simulink model "VK"  (R2022b)
settings: Solver=ode1  StartTime=0.0  StopTime=240  FixedStep=0.01  RelTol=1e-3
undefined symbols (not defined in the file or in its folder): F, Light, MIL, Newton, Raphson, sigbuilder_block
libraries: simulink x3, aerolibwind2 x2, aerolibutil x1, sharedtransform x1
settings Model: Creator=jmira  LastModifiedBy=armando
settings DebuggingCC: UnconnectedInputMsg=warning  UnconnectedOutputMsg=warning  UnconnectedLineMsg=warning
settings ModelReferenceCC: EnableRefExpFcnMdlSchedulingChecks=on
settings RTWCC: DLArmComputeVersion=19.05

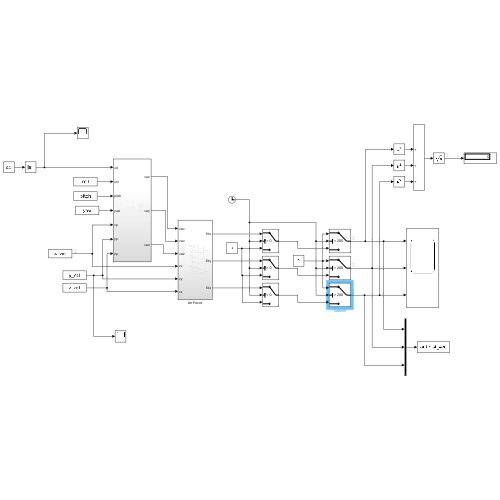
[thumbnail: Simulink's stored preview of the top-level diagram]
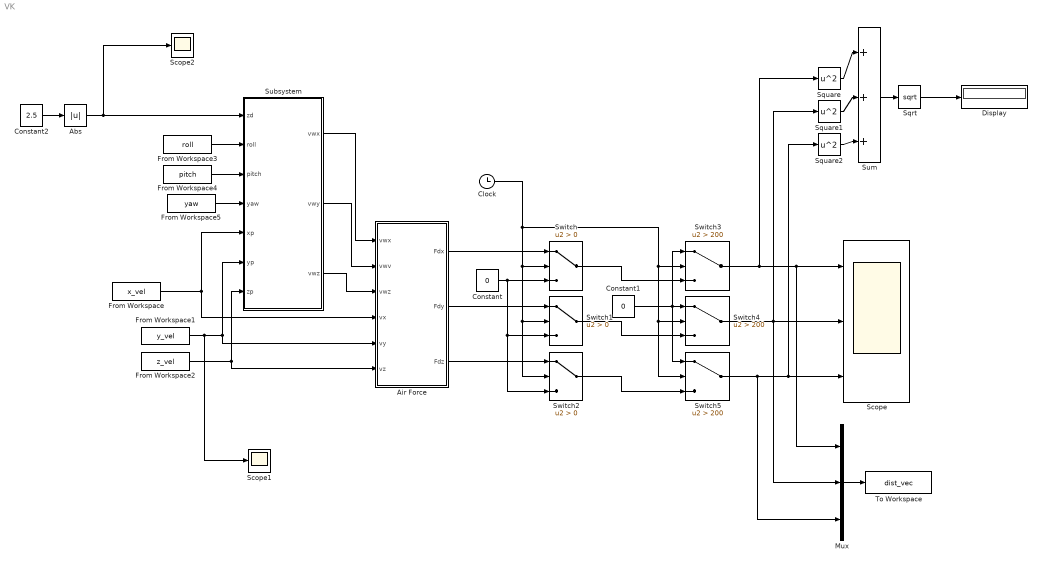
== system VK ==
  Abs : Abs  SaturateOnIntegerOverflow=off
  Air Force : Subsystem
  Clock : Clock
  Constant : Constant  Value=0
  Constant1 : Constant  Value=0
  Constant2 : Constant  Value=2.5
  Display : Display
  From Workspace : FromWorkspace  VariableName=x_vel  SampleTime=0.01
  From Workspace1 : FromWorkspace  VariableName=y_vel  SampleTime=0.01
  From Workspace2 : FromWorkspace  VariableName=z_vel  SampleTime=0.01
  From Workspace3 : FromWorkspace  VariableName=roll  SampleTime=0.01
  From Workspace4 : FromWorkspace  VariableName=pitch  SampleTime=0.01
  From Workspace5 : FromWorkspace  VariableName=yaw  SampleTime=0.01
  Mux : Mux  Inputs=3
  Scope : Scope  NumInputPorts=3
  Scope1 : Scope
  Scope2 : Scope
  Sqrt : Sqrt
  Square : Math  Operator=square
  Square1 : Math  Operator=square
  Square2 : Math  Operator=square
  Subsystem : Subsystem
  Sum : Sum  Inputs=|+++
  Switch : Switch  Criteria=u2 > Threshold  SaturateOnIntegerOverflow=off  InputSameDT=off
  Switch1 : Switch  Criteria=u2 > Threshold  SaturateOnIntegerOverflow=off  InputSameDT=off
  Switch2 : Switch  Criteria=u2 > Threshold  SaturateOnIntegerOverflow=off  InputSameDT=off
  Switch3 : Switch  Criteria=u2 > Threshold  Threshold=200  SaturateOnIntegerOverflow=off  InputSameDT=off
  Switch4 : Switch  Criteria=u2 > Threshold  Threshold=200  SaturateOnIntegerOverflow=off  InputSameDT=off
  Switch5 : Switch  Criteria=u2 > Threshold  Threshold=200  SaturateOnIntegerOverflow=off  InputSameDT=off
  To Workspace : ToWorkspace  VariableName=dist_vec  SampleTime=-1
      settings: Save2DSignal=2-D array (concatenate along first dimension)
  wires:
  Abs/1 -> Scope2/1, Subsystem/1(zd)
  Subsystem/1(vwx) -> Air Force/1(vwx)
  From Workspace/1 -> Air Force/4(vx), Subsystem/5(xp)
  Subsystem/3(vwz) -> Air Force/3(vwz)
  From Workspace1/1 -> Scope1/1, Air Force/5(vy), Subsystem/6(yp)
  Subsystem/2(vwy) -> Air Force/2(vwv)
  From Workspace2/1 -> Air Force/6(vz), Subsystem/7(zp)
  From Workspace3/1 -> Subsystem/2(roll)
  From Workspace4/1 -> Subsystem/3(pitch)
  From Workspace5/1 -> Subsystem/4(yaw)
  Mux/1 -> To Workspace/1
  Air Force/1(Fdx) -> Switch/1
  Clock/1 -> Switch5/2, Switch4/2, Switch3/2, Switch2/2, Switch1/2, Switch/2
  Constant/1 -> Switch2/3, Switch1/3, Switch/3
  Air Force/2(Fdy) -> Switch1/1
  Air Force/3(Fdz) -> Switch2/1
  Switch/1 -> Switch3/3
  Constant1/1 -> Switch5/1, Switch3/1, Switch4/1
  Switch1/1 -> Switch4/3
  Switch2/1 -> Switch5/3
  Switch3/1 -> Square/1, Mux/1, Scope/1
  Switch4/1 -> Square1/1, Mux/2, Scope/2
  Switch5/1 -> Mux/3, Square2/1, Scope/3
  Constant2/1 -> Abs/1
  Square/1 -> Sum/1
  Square2/1 -> Sum/3
  Square1/1 -> Sum/2
  Sum/1 -> Sqrt/1
  Sqrt/1 -> Display/1

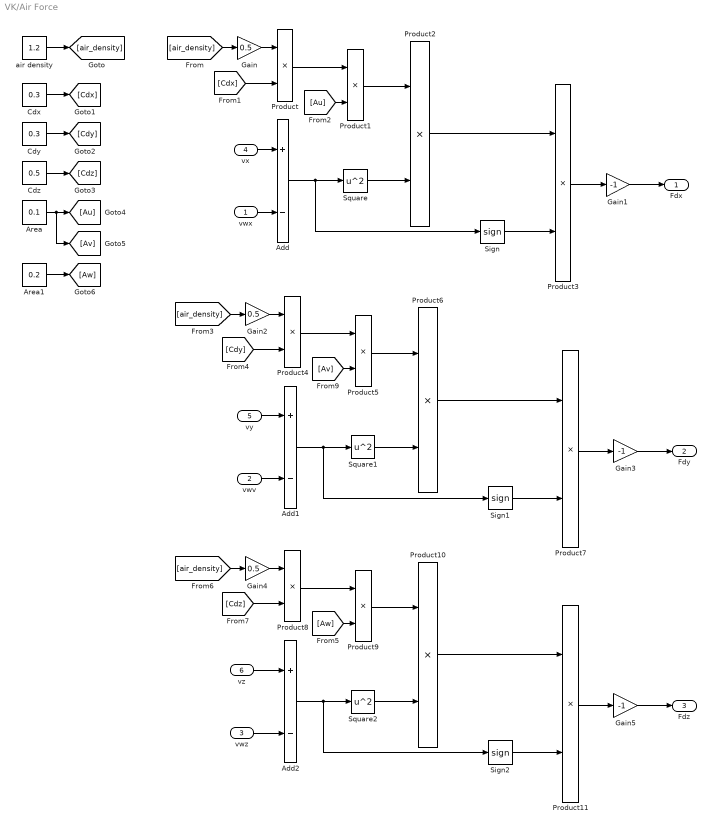
== system VK/Air Force ==
  vwx : Inport
  vwv : Inport  Port=2
  vwz : Inport  Port=3
  vx : Inport  Port=4
  vy : Inport  Port=5
  vz : Inport  Port=6
  Add : Sum  Inputs=+-
  Add1 : Sum  Inputs=+-
  Add2 : Sum  Inputs=+-
  Area : Constant  Value=0.1
  Area1 : Constant  Value=0.2
  Cdx : Constant  Value=0.3
  Cdy : Constant  Value=0.3
  Cdz : Constant  Value=0.5
  Gain : Gain  Gain=0.5
  Gain1 : Gain  Gain=-1
  Gain2 : Gain  Gain=0.5
  Gain3 : Gain  Gain=-1
  Gain4 : Gain  Gain=0.5
  Gain5 : Gain  Gain=-1
  Product{,1..11} (12 alike) : Product
  Sign : Signum
  Sign1 : Signum
  Sign2 : Signum
  Square : Math  Operator=square
  Square1 : Math  Operator=square
  Square2 : Math  Operator=square
  air density : Constant  Value=1.2
  Fdx : Outport
  Fdy : Outport  Port=2
  Fdz : Outport  Port=3
  wires:
  air density/1 -> [air_density]
  [air_density] -> Gain/1
  Cdx/1 -> [Cdx]
  Cdy/1 -> [Cdy]
  Cdz/1 -> [Cdz]
  Gain/1 -> Product/1
  [Cdx] -> Product/2
  Area/1 -> [Av], [Au]
  Product/1 -> Product1/1
  [Au] -> Product1/2
  Product1/1 -> Product2/1
  Square/1 -> Product2/2
  Add/1 -> Sign/1, Square/1
  vx/1 -> Add/1
  vwx/1 -> Add/2
  Product2/1 -> Product3/1
  Sign/1 -> Product3/2
  Product3/1 -> Gain1/1
  Gain1/1 -> Fdx/1
  Gain3/1 -> Fdy/1
  Product7/1 -> Gain3/1
  Sign1/1 -> Product7/2
  Product6/1 -> Product7/1
  vwv/1 -> Add1/2
  vy/1 -> Add1/1
  Add1/1 -> Square1/1, Sign1/1
  Square1/1 -> Product6/2
  Product5/1 -> Product6/1
  [Av] -> Product5/2
  Product4/1 -> Product5/1
  [Cdy] -> Product4/2
  Gain2/1 -> Product4/1
  [air_density] -> Gain2/1
  [air_density] -> Gain4/1
  Gain4/1 -> Product8/1
  [Cdz] -> Product8/2
  Product8/1 -> Product9/1
  [Aw] -> Product9/2
  Product9/1 -> Product10/1
  Square2/1 -> Product10/2
  Add2/1 -> Sign2/1, Square2/1
  Product10/1 -> Product11/1
  Sign2/1 -> Product11/2
  Product11/1 -> Gain5/1
  Gain5/1 -> Fdz/1
  vz/1 -> Add2/1
  vwz/1 -> Add2/2
  Area1/1 -> [Aw]

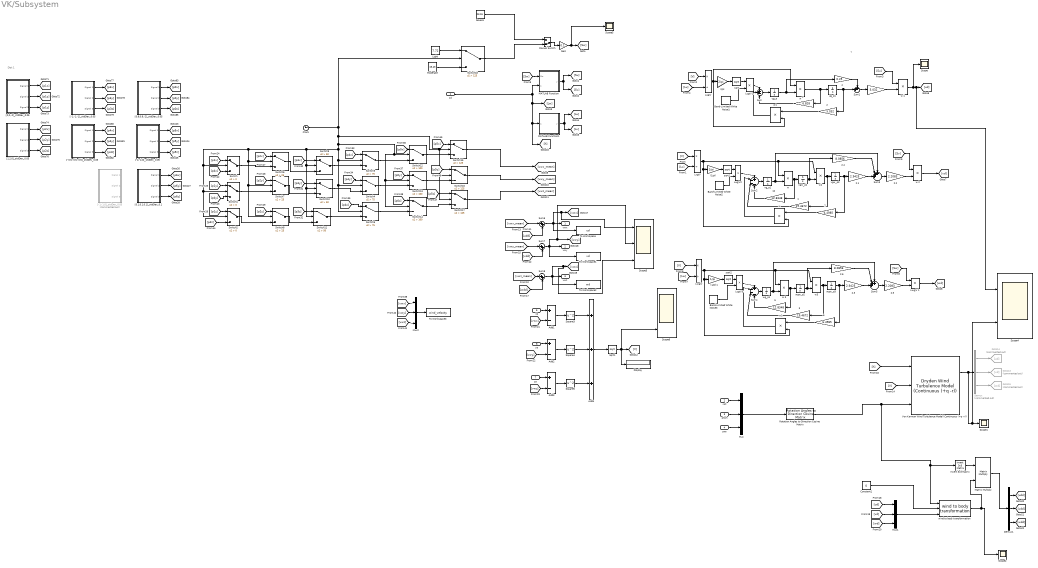
== system VK/Subsystem ==
  note: u
  note: Dist 1
  zd : Inport
  roll : Inport  Port=2
  pitch : Inport  Port=3
  yaw : Inport  Port=4
  xp : Inport  Port=5
  yp : Inport  Port=6
  zp : Inport  Port=7
  " " : Gain  Gain=5.032  SaturateOnIntegerOverflow=on  OutDataTypeStr=Inherit: Same as input  ParamDataTypeStr=Inherit: Same as input
  " 1" : Gain  Gain=6.828  SaturateOnIntegerOverflow=on  OutDataTypeStr=Inherit: Same as input  ParamDataTypeStr=Inherit: Same as input
  " 2" : Gain  Gain=5.032  SaturateOnIntegerOverflow=on  OutDataTypeStr=Inherit: Same as input  ParamDataTypeStr=Inherit: Same as input
  " w" : Product  InputSameDT=on  SaturateOnIntegerOverflow=on  OutDataTypeStr=Inherit: Same as first input
  " w1" : Product  InputSameDT=on  SaturateOnIntegerOverflow=on  OutDataTypeStr=Inherit: Same as first input
  (1/pi) : Gain  Gain=1/pi  SaturateOnIntegerOverflow=on  OutDataTypeStr=Inherit: Same as input  ParamDataTypeStr=Inherit: Same as input
  (1/pi)1 : Gain  Gain=1/pi  SaturateOnIntegerOverflow=on  OutDataTypeStr=Inherit: Same as input  ParamDataTypeStr=Inherit: Same as input
  1 : Gain  Gain=19.4672  SaturateOnIntegerOverflow=on  OutDataTypeStr=Inherit: Same as input  ParamDataTypeStr=Inherit: Same as input
  12 : Gain  Gain=12.8348  SaturateOnIntegerOverflow=on  OutDataTypeStr=Inherit: Same as input  ParamDataTypeStr=Inherit: Same as input
  2 : Gain  Gain=6.4985  SaturateOnIntegerOverflow=on  OutDataTypeStr=Inherit: Same as input  ParamDataTypeStr=Inherit: Same as input
  2.1 : Gain  Gain=2.9425  SaturateOnIntegerOverflow=on  OutDataTypeStr=Inherit: Same as input  ParamDataTypeStr=Inherit: Same as input
  2.2 : Gain  Gain=2.2083  SaturateOnIntegerOverflow=on  OutDataTypeStr=Inherit: Same as input  ParamDataTypeStr=Inherit: Same as input
  2.3 : Gain  Gain=2.9425  SaturateOnIntegerOverflow=on  OutDataTypeStr=Inherit: Same as input  ParamDataTypeStr=Inherit: Same as input
  2.4 : Gain  Gain=8.0856  SaturateOnIntegerOverflow=on  OutDataTypeStr=Inherit: Same as input  ParamDataTypeStr=Inherit: Same as input
  2.5 : Gain  Gain=2.2083  SaturateOnIntegerOverflow=on  OutDataTypeStr=Inherit: Same as input  ParamDataTypeStr=Inherit: Same as input
  2.6 : Gain  Gain=8.0856  SaturateOnIntegerOverflow=on  OutDataTypeStr=Inherit: Same as input  ParamDataTypeStr=Inherit: Same as input
  2/pi : Gain  Gain=2/pi  SaturateOnIntegerOverflow=on  OutDataTypeStr=Inherit: Same as input  ParamDataTypeStr=Inherit: Same as input
  3 : Gain  Gain=19.4672  SaturateOnIntegerOverflow=on  OutDataTypeStr=Inherit: Same as input  ParamDataTypeStr=Inherit: Same as input
  4 : Gain  Gain=0.25  SaturateOnIntegerOverflow=on  OutDataTypeStr=Inherit: Same as input  ParamDataTypeStr=Inherit: Same as input
  5 : Gain  Gain=12.8348  SaturateOnIntegerOverflow=on  OutDataTypeStr=Inherit: Same as input  ParamDataTypeStr=Inherit: Same as input
  6 : Gain  Gain=6.4985  SaturateOnIntegerOverflow=on  OutDataTypeStr=Inherit: Same as input  ParamDataTypeStr=Inherit: Same as input
  Add1 : Sum  Inputs=+-
  Add2 : Sum  Inputs=+-
  Add3 : Sum  Inputs=+-
  Add4 : Sum  Inputs=+++
  Band-Limited White Noise1 : simulink/Sources/Band-Limited White Noise  Cov=3  Ts=0.1  seed=[23341]
  Band-Limited White Noise2 : simulink/Sources/Band-Limited White Noise  Cov=3  Ts=0.1  seed=[23342]
  Band-Limited White Noise3 : simulink/Sources/Band-Limited White Noise  Cov=3  Ts=0.1  seed=[23343]
  Clock : Clock
  Constant1 : Constant  Value=0
  Demux : Demux  Commented=on  Outputs=3
  Demux1 : Demux  Outputs=3
  Display : Display
  Gain : Gain  Gain=0.1
  Goto13 : Goto  Commented=on  GotoTag=vd
  Goto14 : Goto  Commented=on  GotoTag=ud
  Goto15 : Goto  Commented=on  GotoTag=wd
  Invert 3x3 Matrix : aerolibutil/Invert  3x3 Matrix
  Light : Constant  Value=7.72
  Lug/V : Product  Inputs=*/  InputSameDT=on  SaturateOnIntegerOverflow=on  OutDataTypeStr=Inherit: Same as first input
  Lug/V1 : Product  InputSameDT=on  SaturateOnIntegerOverflow=on  OutDataTypeStr=Inherit: Same as first input
  Lug/V2 : Product  InputSameDT=on  SaturateOnIntegerOverflow=on  OutDataTypeStr=Inherit: Same as first input
  Lug/V3 : Product  InputSameDT=on  SaturateOnIntegerOverflow=on  OutDataTypeStr=Inherit: Same as first input
  Lvg/V : Product  Inputs=*/  InputSameDT=on  SaturateOnIntegerOverflow=on  OutDataTypeStr=Inherit: Same as first input
  Lwg/V : Product  Inputs=*/  InputSameDT=on  SaturateOnIntegerOverflow=on  OutDataTypeStr=Inherit: Same as first input
  Lwg/V 1 : Product  InputSameDT=on  SaturateOnIntegerOverflow=on  OutDataTypeStr=Inherit: Same as first input
  MATLAB Function : MATLAB Function  TreatAsAtomicUnit=on
  MATLAB Function1 : MATLAB Function  TreatAsAtomicUnit=on
  Manual Switch : ManualSwitch  CurrentSetting=0
  Matrix Multiply : Product  Multiplication=Matrix(*)
  Moderate : Constant  Value=15.43
  Mux : Mux  Inputs=3
  Mux1 : Mux  Inputs=3
  Mux2 : Mux  Inputs=3
  Rotation Angles to Direction Cosine Matrix : sharedtransform/Rotation Angles to Direction Cosine Matrix  rotationOrder=ZYX  aMode=aMode
  Scope{,1..2,5} (4 alike) : Scope
  Scope3 : Scope  NumInputPorts=3
  Scope4 : Scope  NumInputPorts=2
  Scope6 : Scope  NumInputPorts=3
  Severe : Constant  Value=23.15
  Sqrt1 : Sqrt
  Square3 : Math  Operator=square
  Square4 : Math  Operator=square
  Square5 : Math  Operator=square
  Sum : Sum  Inputs=+--  InputSameDT=on  SaturateOnIntegerOverflow=on  OutDataTypeStr=Inherit: Same as first input
  Sum1 : Sum  Inputs=++|  InputSameDT=on  SaturateOnIntegerOverflow=on  OutDataTypeStr=Inherit: Same as first input
  Sum2 : Sum  Inputs=+---  InputSameDT=on  SaturateOnIntegerOverflow=on  OutDataTypeStr=Inherit: Same as first input
  Sum3 : Sum  Inputs=+++||  InputSameDT=on  SaturateOnIntegerOverflow=on  OutDataTypeStr=Inherit: Same as first input
  Sum4 : Sum  Inputs=+---  InputSameDT=on  SaturateOnIntegerOverflow=on  OutDataTypeStr=Inherit: Same as first input
  Sum5 : Sum  Inputs=+++||  InputSameDT=on  SaturateOnIntegerOverflow=on  OutDataTypeStr=Inherit: Same as first input
  Sum6 : Sum  Inputs=|++
  Sum7 : Sum  Inputs=|++
  Sum8 : Sum  Inputs=|++
  Switch : Switch  Criteria=u2 > Threshold  SaturateOnIntegerOverflow=off  InputSameDT=off
  Switch1 : Switch  Criteria=u2 > Threshold  SaturateOnIntegerOverflow=off  InputSameDT=off
  Switch10 : Switch  Criteria=u2 > Threshold  Threshold=50  SaturateOnIntegerOverflow=off  InputSameDT=off
  Switch11 : Switch  Criteria=u2 > Threshold  Threshold=50  SaturateOnIntegerOverflow=off  InputSameDT=off
  Switch12 : Switch  Criteria=u2 > Threshold  Threshold=100  SaturateOnIntegerOverflow=off  InputSameDT=off
  Switch13 : Switch  Criteria=u2 > Threshold  Threshold=100  SaturateOnIntegerOverflow=off  InputSameDT=off
  Switch14 : Switch  Criteria=u2 > Threshold  Threshold=100  SaturateOnIntegerOverflow=off  InputSameDT=off
  Switch{15..18} (4 alike) : Switch  Criteria=u2 > Threshold  Threshold=125  SaturateOnIntegerOverflow=off  InputSameDT=off
  Switch2 : Switch  Criteria=u2 > Threshold  SaturateOnIntegerOverflow=off  InputSameDT=off
  Switch3 : Switch  Criteria=u2 > Threshold  Threshold=75  SaturateOnIntegerOverflow=off  InputSameDT=off
  Switch4 : Switch  Criteria=u2 > Threshold  Threshold=75  SaturateOnIntegerOverflow=off  InputSameDT=off
  Switch5 : Switch  Criteria=u2 > Threshold  Threshold=75  SaturateOnIntegerOverflow=off  InputSameDT=off
  Switch6 : Switch  Criteria=u2 > Threshold  Threshold=25  SaturateOnIntegerOverflow=off  InputSameDT=off
  Switch7 : Switch  Criteria=u2 > Threshold  Threshold=25  SaturateOnIntegerOverflow=off  InputSameDT=off
  Switch8 : Switch  Criteria=u2 > Threshold  Threshold=25  SaturateOnIntegerOverflow=off  InputSameDT=off
  Switch9 : Switch  Criteria=u2 > Threshold  Threshold=50  SaturateOnIntegerOverflow=off  InputSameDT=off
  To Workspace : ToWorkspace  VariableName=ud  SampleTime=-1
      settings: Save2DSignal=2-D array (concatenate along first dimension)
  To Workspace1 : ToWorkspace  VariableName=vd  SampleTime=-1
      settings: Save2DSignal=2-D array (concatenate along first dimension)
  To Workspace2 : ToWorkspace  VariableName=wd  SampleTime=-1
      settings: Save2DSignal=2-D array (concatenate along first dimension)
  To Workspace3 : ToWorkspace  VariableName=wind_velocity  SampleTime=-1
      settings: Save2DSignal=2-D array (concatenate along first dimension)
  Von Karman Wind Turbulence Model (Continuous (+q -r)) : aerolibwind2/Dryden Wind Turbulence Model  (Continuous (+q -r))  units=Metric (MKS)  spec=MIL-F-8785C  model=Continuous Von Karman (+q +r)  W20=15  Wdeg=0  TurbProb=10^-2 - Light  L_high=762  Wingspan=0.5  ts=0.1  Seed=[23341 23342 23343 23344]  T_on=on
  "[-0.5,-0.5,-0.5]_stdDev_0.05" : Subsystem  Tag=STV Subsys  LoadFcn=sigbuilder_block('load');  StartFcn=sigbuilder_block('start');  StopFcn=sigbuilder_block('stop');  ClipboardFcn=sigbuilder_block('clipboard');  mask(Sigbuilder block){tuvar=[0:10]}
      mask help: Simulink:masks:SigbuilderBlock_MD
      mask init:
      | if ~strcmp(get_param(bdroot(gcbh),'SimulationStatus'),'stopped') tuvar = sigbuilder_block('maskInit'); end
      settings: CopyFcn=sigbuilder_block('copy');  DeleteFcn=sigbuilder_block('delete');  ModelCloseFcn=sigbuilder_block('modelClose');  PreSaveFcn=sigbuilder_block('preSave');  PauseFcn=sigbuilder_block('pause');  ContinueFcn=sigbuilder_block('continue');  NameChangeFcn=sigbuilder_block('namechange');  OpenFcn=sigbuilder_block('open',[750.75 81.75 549.75 399.75 ]);  CloseFcn=sigbuilder_block('close');
      mask Display: plot(0, 0, 100, 100,[2, 2, 32, 32, 2], [68, 8, 8, 68, 68],[32, 2], [38, 38], [32, 19, 2],[53, 60, 44], [32, 17, 17, 2],[16, 16, 31, 31]);txt = getActiveGroup(gcbh);text(2, 100, txt,'verticalAlignment', 'top');
  "[-1,-1,-1]_stdDev_0.05" : Subsystem  Tag=STV Subsys  LoadFcn=sigbuilder_block('load');  StartFcn=sigbuilder_block('start');  StopFcn=sigbuilder_block('stop');  ClipboardFcn=sigbuilder_block('clipboard');  mask(Sigbuilder block){tuvar=[0:10]}
      mask help: Simulink:masks:SigbuilderBlock_MD
      mask init:
      | if ~strcmp(get_param(bdroot(gcbh),'SimulationStatus'),'stopped') tuvar = sigbuilder_block('maskInit'); end
      settings: CopyFcn=sigbuilder_block('copy');  DeleteFcn=sigbuilder_block('delete');  ModelCloseFcn=sigbuilder_block('modelClose');  PreSaveFcn=sigbuilder_block('preSave');  PauseFcn=sigbuilder_block('pause');  ContinueFcn=sigbuilder_block('continue');  NameChangeFcn=sigbuilder_block('namechange');  OpenFcn=sigbuilder_block('open',[786.75 219.75 550.5 399.75 ]);  CloseFcn=sigbuilder_block('close');
      mask Display: plot(0, 0, 100, 100,[2, 2, 32, 32, 2], [68, 8, 8, 68, 68],[32, 2], [38, 38], [32, 19, 2],[53, 60, 44], [32, 17, 17, 2],[16, 16, 31, 31]);txt = getActiveGroup(gcbh);text(2, 100, txt,'verticalAlignment', 'top');
  "[-1,-1,0]_stdDev_0.05" : Subsystem  Tag=STV Subsys  Commented=on  LoadFcn=sigbuilder_block('load');  StartFcn=sigbuilder_block('start');  StopFcn=sigbuilder_block('stop');  ClipboardFcn=sigbuilder_block('clipboard');  mask(Sigbuilder block){tuvar=[0:10]}
      mask help: Simulink:masks:SigbuilderBlock_MD
      mask init:
      | if ~strcmp(get_param(bdroot(gcbh),'SimulationStatus'),'stopped') tuvar = sigbuilder_block('maskInit'); end
      settings: CopyFcn=sigbuilder_block('copy');  DeleteFcn=sigbuilder_block('delete');  ModelCloseFcn=sigbuilder_block('modelClose');  PreSaveFcn=sigbuilder_block('preSave');  PauseFcn=sigbuilder_block('pause');  ContinueFcn=sigbuilder_block('continue');  NameChangeFcn=sigbuilder_block('namechange');  OpenFcn=sigbuilder_block('open',[253.5 0 610.5 357.75 ]);  CloseFcn=sigbuilder_block('close');
      mask Display: plot(0, 0, 100, 100,[2, 2, 32, 32, 2], [68, 8, 8, 68, 68],[32, 2], [38, 38], [32, 19, 2],[53, 60, 44], [32, 17, 17, 2],[16, 16, 31, 31]);txt = getActiveGroup(gcbh);text(2, 100, txt,'verticalAlignment', 'top');
  "[-2,-2,0]_stdDev_0.05" : Subsystem  Tag=STV Subsys  LoadFcn=sigbuilder_block('load');  StartFcn=sigbuilder_block('start');  StopFcn=sigbuilder_block('stop');  ClipboardFcn=sigbuilder_block('clipboard');  mask(Sigbuilder block){tuvar=[0:10]}
      mask help: Simulink:masks:SigbuilderBlock_MD
      mask init:
      | if ~strcmp(get_param(bdroot(gcbh),'SimulationStatus'),'stopped') tuvar = sigbuilder_block('maskInit'); end
      settings: CopyFcn=sigbuilder_block('copy');  DeleteFcn=sigbuilder_block('delete');  ModelCloseFcn=sigbuilder_block('modelClose');  PreSaveFcn=sigbuilder_block('preSave');  PauseFcn=sigbuilder_block('pause');  ContinueFcn=sigbuilder_block('continue');  NameChangeFcn=sigbuilder_block('namechange');  OpenFcn=sigbuilder_block('open',[238.5 0 633 342 ]);  CloseFcn=sigbuilder_block('close');
      mask Display: plot(0, 0, 100, 100,[2, 2, 32, 32, 2], [68, 8, 8, 68, 68],[32, 2], [38, 38], [32, 19, 2],[53, 60, 44], [32, 17, 17, 2],[16, 16, 31, 31]);txt = getActiveGroup(gcbh);text(2, 100, txt,'verticalAlignment', 'top');
  "[0,0,-2]_stdDev_0.05" : Subsystem  Tag=STV Subsys  LoadFcn=sigbuilder_block('load');  StartFcn=sigbuilder_block('start');  StopFcn=sigbuilder_block('stop');  ClipboardFcn=sigbuilder_block('clipboard');  mask(Sigbuilder block){tuvar=[0:10]}
      mask help: Simulink:masks:SigbuilderBlock_MD
      mask init:
      | if ~strcmp(get_param(bdroot(gcbh),'SimulationStatus'),'stopped') tuvar = sigbuilder_block('maskInit'); end
      settings: CopyFcn=sigbuilder_block('copy');  DeleteFcn=sigbuilder_block('delete');  ModelCloseFcn=sigbuilder_block('modelClose');  PreSaveFcn=sigbuilder_block('preSave');  PauseFcn=sigbuilder_block('pause');  ContinueFcn=sigbuilder_block('continue');  NameChangeFcn=sigbuilder_block('namechange');  OpenFcn=sigbuilder_block('open',[783 195.75 550.5 399.75 ]);  CloseFcn=sigbuilder_block('close');
      mask Display: plot(0, 0, 100, 100,[2, 2, 32, 32, 2], [68, 8, 8, 68, 68],[32, 2], [38, 38], [32, 19, 2],[53, 60, 44], [32, 17, 17, 2],[16, 16, 31, 31]);txt = getActiveGroup(gcbh);text(2, 100, txt,'verticalAlignment', 'top');
  "[0.1,0.1,0.1]_stdDev_0.1" : Subsystem  Tag=STV Subsys  LoadFcn=sigbuilder_block('load');  StartFcn=sigbuilder_block('start');  StopFcn=sigbuilder_block('stop');  ClipboardFcn=sigbuilder_block('clipboard');  mask(Sigbuilder block){tuvar=[0:10]}
      mask help: Simulink:masks:SigbuilderBlock_MD
      mask init:
      | if ~strcmp(get_param(bdroot(gcbh),'SimulationStatus'),'stopped') tuvar = sigbuilder_block('maskInit'); end
      settings: CopyFcn=sigbuilder_block('copy');  DeleteFcn=sigbuilder_block('delete');  ModelCloseFcn=sigbuilder_block('modelClose');  PreSaveFcn=sigbuilder_block('preSave');  PauseFcn=sigbuilder_block('pause');  ContinueFcn=sigbuilder_block('continue');  NameChangeFcn=sigbuilder_block('namechange');  OpenFcn=sigbuilder_block('open',[429.75 180.75 550.5 399.75 ]);  CloseFcn=sigbuilder_block('close');
      mask Display: plot(0, 0, 100, 100,[2, 2, 32, 32, 2], [68, 8, 8, 68, 68],[32, 2], [38, 38], [32, 19, 2],[53, 60, 44], [32, 17, 17, 2],[16, 16, 31, 31]);txt = getActiveGroup(gcbh);text(2, 100, txt,'verticalAlignment', 'top');
  "[0.8,0.8,-2]_stdDev_0.05" : Subsystem  Tag=STV Subsys  LoadFcn=sigbuilder_block('load');  StartFcn=sigbuilder_block('start');  StopFcn=sigbuilder_block('stop');  ClipboardFcn=sigbuilder_block('clipboard');  mask(Sigbuilder block){tuvar=[0:10]}
      mask help: Simulink:masks:SigbuilderBlock_MD
      mask init:
      | if ~strcmp(get_param(bdroot(gcbh),'SimulationStatus'),'stopped') tuvar = sigbuilder_block('maskInit'); end
      settings: CopyFcn=sigbuilder_block('copy');  DeleteFcn=sigbuilder_block('delete');  ModelCloseFcn=sigbuilder_block('modelClose');  PreSaveFcn=sigbuilder_block('preSave');  PauseFcn=sigbuilder_block('pause');  ContinueFcn=sigbuilder_block('continue');  NameChangeFcn=sigbuilder_block('namechange');  OpenFcn=sigbuilder_block('open',[426 183 565.5 389.25 ]);  CloseFcn=sigbuilder_block('close');
      mask Display: plot(0, 0, 100, 100,[2, 2, 32, 32, 2], [68, 8, 8, 68, 68],[32, 2], [38, 38], [32, 19, 2],[53, 60, 44], [32, 17, 17, 2],[16, 16, 31, 31]);txt = getActiveGroup(gcbh);text(2, 100, txt,'verticalAlignment', 'top');
  "[2,2,0]_stdDev_0.05" : Subsystem  Tag=STV Subsys  LoadFcn=sigbuilder_block('load');  StartFcn=sigbuilder_block('start');  StopFcn=sigbuilder_block('stop');  ClipboardFcn=sigbuilder_block('clipboard');  mask(Sigbuilder block){tuvar=[0:10]}
      mask help: Simulink:masks:SigbuilderBlock_MD
      mask init:
      | if ~strcmp(get_param(bdroot(gcbh),'SimulationStatus'),'stopped') tuvar = sigbuilder_block('maskInit'); end
      settings: CopyFcn=sigbuilder_block('copy');  DeleteFcn=sigbuilder_block('delete');  ModelCloseFcn=sigbuilder_block('modelClose');  PreSaveFcn=sigbuilder_block('preSave');  PauseFcn=sigbuilder_block('pause');  ContinueFcn=sigbuilder_block('continue');  NameChangeFcn=sigbuilder_block('namechange');  OpenFcn=sigbuilder_block('open',[766.5 217.5 550.5 399.75 ]);  CloseFcn=sigbuilder_block('close');
      mask Display: plot(0, 0, 100, 100,[2, 2, 32, 32, 2], [68, 8, 8, 68, 68],[32, 2], [38, 38], [32, 19, 2],[53, 60, 44], [32, 17, 17, 2],[16, 16, 31, 31]);txt = getActiveGroup(gcbh);text(2, 100, txt,'verticalAlignment', 'top');
  sqrt : Sqrt  AlgorithmType=Newton-Raphson
  sqrt1 : Sqrt  AlgorithmType=Newton-Raphson
  sqrt2 : Sqrt  AlgorithmType=Newton-Raphson
  ug_p : Integrator
  ug_p1 : Integrator
  vg_p1 : Integrator
  vgw_p2 : Integrator
  vgw_p3 : Integrator
  w{,1..3} (4 alike) : Product  InputSameDT=on  SaturateOnIntegerOverflow=on  OutDataTypeStr=Inherit: Same as first input
  w {,1..3} (4 alike) : Product  InputSameDT=on  SaturateOnIntegerOverflow=on  OutDataTypeStr=Inherit: Same as first input
  wg_p1 : Integrator
  wgw_p2 : Integrator
  wgw_p3 : Integrator
  wind to body transformation : aerolibwind2/Dryden Wind Turbulence Model  (Continuous (+q -r))/Select velocities/Low altitude  velocities/wind to body transformation  SystemSampleTime=-1  VariantActivationTime=update diagram  Latency=0  AutoFrameSizeCalculation=off
  vwx : Outport
  vwy : Outport  Port=2
  vwz : Outport  Port=3
  wires:
  [Lu] -> Lug/V/2
  Band-Limited White Noise3/1 -> Lug/V3/2
  Band-Limited White Noise2/1 -> Lug/V2/2
  [Sv] -> w 2/1
  Lug/V2/1 -> Sum2/1
  Lvg/V/1 -> "w "/1, w2/1, (1/pi)/1, " w"/2
  sqrt1/1 -> Lug/V2/1
  vg_p1/1 -> "w "/2, Sum3/1
  (1/pi)/1 -> sqrt1/1
  "w "/1 -> 12/1, vgw_p2/1
  vgw_p2/1 -> w2/2, 2.4/1
  Sum2/1 -> vg_p1/1
  2/1 -> " w"/1
  2.1/1 -> Sum3/3
  2.2/1 -> w 2/2
  Sum3/1 -> 2.2/1
  [Lv] -> Lvg/V/2
  " w"/1 -> Sum2/2
  1/1 -> Sum2/3
  vgw_p3/1 -> 2/1, 2.1/1
  2.4/1 -> Sum3/2
  [Su] -> w 1/1
  ug_p1/1 -> " 2"/1, Sum1/2
  Lug/V/1 -> 2/pi/1, w1/2, w/1
  Band-Limited White Noise1/1 -> Lug/V1/2
  [Sw] -> Lwg/V 1/1
  wg_p1/1 -> w 3/2, Sum5/1
  (1/pi)1/1 -> sqrt2/1
  wgw_p2/1 -> w3/2, 2.6/1
  2/pi/1 -> sqrt/1
  5/1 -> Sum4/4
  Sum5/1 -> 2.5/1
  6/1 -> " w1"/1
  w3/1 -> 3/1, wgw_p3/1
  12/1 -> Sum2/4
  3/1 -> Sum4/3
  wgw_p3/1 -> 6/1, 2.3/1
  " w1"/1 -> Sum4/2
  2.5/1 -> Lwg/V 1/2
  Lug/V1/1 -> Sum/1
  w2/1 -> 1/1, vgw_p3/1
  2.6/1 -> Sum5/2
  ug_p/1 -> 4/1, w/2
  Sum1/1 -> " "/1
  sqrt2/1 -> Lug/V3/1
  Lwg/V/1 -> (1/pi)1/1, " w1"/2, w 3/1, w3/1
  Sum/1 -> ug_p/1
  [Lw] -> Lwg/V/2
  " 2"/1 -> w1/1
  " "/1 -> w 1/2
  w 3/1 -> 5/1, wgw_p2/1
  2.3/1 -> Sum5/3
  sqrt/1 -> Lug/V1/1
  4/1 -> Sum1/1
  " 1"/1 -> Sum/3
  w/1 -> ug_p1/1, " 1"/1
  Sum4/1 -> wg_p1/1
  w1/1 -> Sum/2
  Lug/V3/1 -> Sum4/1
  Gain/1 -> Scope5/1, [Sw]
  [Sw] -> MATLAB Function/1(Sw)
  MATLAB Function/1(y) -> [Sv], [Su]
  MATLAB Function1/1(y) -> [Lv], [Lu]
  Lwg/V 1/1 -> [wd]
  [vwx_mean] -> Sum6/1
  Sum6/1 -> Scope3/1, [vwx], vwx/1, To Workspace/1
  [vwy_mean] -> Sum7/1
  zd/1 -> MATLAB Function/2(z), [h], MATLAB Function1/1(z), [Lw]
  Von Karman Wind Turbulence Model (Continuous (+q -r))/1 -> Scope4/2, Scope1/1, Demux/1
  Demux/1 -> Goto14/1
  Demux/2 -> Goto13/1
  Demux/3 -> Goto15/1
  Mux/1 -> Rotation Angles to Direction Cosine Matrix/1
  roll/1 -> Mux/1
  pitch/1 -> Mux/2
  yaw/1 -> Mux/3
  xp/1 -> Add1/1
  yp/1 -> Add2/1
  zp/1 -> Add3/1
  Add1/1 -> Square3/1
  Add2/1 -> Square4/1
  Add3/1 -> Square5/1
  Square5/1 -> Add4/3
  Square4/1 -> Add4/2
  Square3/1 -> Add4/1
  Sqrt1/1 -> Scope6/3, Display/1, [V]
  [V] -> Lwg/V/1
  [V] -> Lvg/V/1
  [h] -> Von Karman Wind Turbulence Model (Continuous (+q -r))/1
  Add4/1 -> Sqrt1/1
  [vwz_mean] -> Sum8/1
  [wdd] -> Sum8/2
  [vdd] -> Sum7/2
  [udd] -> Sum6/2
  [V] -> Von Karman Wind Turbulence Model (Continuous (+q -r))/2
  Sum7/1 -> [vwy], Scope3/2, To Workspace1/1, vwy/1
  Sum8/1 -> Scope3/3, [vwz], vwz/1, To Workspace2/1
  [V] -> Lug/V/1
  w 1/1 -> Scope/1, Scope4/1, [ud]
  Rotation Angles to Direction Cosine Matrix/1 -> Invert 3x3 Matrix/1, wind to body transformation/1, Von Karman Wind Turbulence Model (Continuous (+q -r))/3
  [ud] -> Mux1/1
  [wd] -> Mux1/3
  Mux1/1 -> wind to body transformation/3
  Constant1/1 -> wind to body transformation/2
  wind to body transformation/1 -> Matrix Multiply/2, Scope2/1
  [vd] -> Mux1/2
  Demux1/1 -> [udd]
  Demux1/2 -> [vdd]
  Demux1/3 -> [wdd]
  w 2/1 -> [vd]
  Invert 3x3 Matrix/1 -> Matrix Multiply/1
  Matrix Multiply/1 -> Demux1/1
  [vwx] -> Add1/2
  [vwy] -> Add2/2
  [vwz] -> Add3/2
  Severe/1 -> Manual Switch/1
  Manual Switch/1 -> Gain/1
  [p4x] -> Switch/3
  [p4y] -> Switch1/3
  [p4z] -> Switch2/3
  [p4x] -> Switch3/1
  [p4y] -> Switch4/1
  [p4z] -> Switch5/1
  Switch/1 -> Switch6/3
  Switch1/1 -> Switch7/3
  Switch2/1 -> Switch8/3
  Switch9/1 -> Switch3/3
  Switch6/1 -> Switch9/3
  [p3x] -> Switch9/1
  Switch10/1 -> Switch4/3
  Switch7/1 -> Switch10/3
  [p3y] -> Switch10/1
  Switch11/1 -> Switch5/3
  Switch8/1 -> Switch11/3
  [p3z] -> Switch11/1
  [p2x] -> Switch6/1
  [p1x] -> Switch/1
  [p2y] -> Switch7/1
  [p1y] -> Switch1/1
  [p2z] -> Switch8/1
  [p1z] -> Switch2/1
  [vwx] -> Mux2/1
  [vwy] -> Mux2/2
  [vwz] -> Mux2/3
  Mux2/1 -> To Workspace3/1
  "[0,0,-2]_stdDev_0.05"/1(Signal 1) -> [p1x]
  "[0,0,-2]_stdDev_0.05"/2(Signal 2) -> [p1y]
  "[0,0,-2]_stdDev_0.05"/3(Signal 3) -> [p1z]
  "[-0.5,-0.5,-0.5]_stdDev_0.05"/3(Signal 3) -> [p4z]
  "[-0.5,-0.5,-0.5]_stdDev_0.05"/2(Signal 2) -> [p4y]
  "[-0.5,-0.5,-0.5]_stdDev_0.05"/1(Signal 1) -> [p4x]
  "[0.8,0.8,-2]_stdDev_0.05"/1(Signal 1) -> [p0x]
  "[0.8,0.8,-2]_stdDev_0.05"/2(Signal 2) -> [p0y]
  "[0.8,0.8,-2]_stdDev_0.05"/3(Signal 3) -> [p0z]
  "[-1,-1,-1]_stdDev_0.05"/1(Signal 1) -> [p3x]
  "[-1,-1,-1]_stdDev_0.05"/2(Signal 2) -> [p3y]
  "[-1,-1,-1]_stdDev_0.05"/3(Signal 3) -> [p3z]
  "[2,2,0]_stdDev_0.05"/1(Signal 1) -> [p2x]
  "[2,2,0]_stdDev_0.05"/2(Signal 2) -> [p2y]
  "[2,2,0]_stdDev_0.05"/3(Signal 3) -> [p2z]
  Switch3/1 -> Switch12/3
  Switch4/1 -> Switch13/3
  Switch5/1 -> Switch14/3
  [p0x] -> Switch12/1
  [p0y] -> Switch13/1
  [p0z] -> Switch14/1
  Switch12/1 -> Switch15/3
  Switch13/1 -> Switch16/3
  Switch14/1 -> Switch17/3
  "[-2,-2,0]_stdDev_0.05"/2(Signal 2) -> [p5y]
  "[-2,-2,0]_stdDev_0.05"/3(Signal 3) -> [p5z]
  "[-2,-2,0]_stdDev_0.05"/1(Signal 1) -> [p5x]
  [p5x] -> Switch15/1
  [p5y] -> Switch16/1
  [p5z] -> Switch17/1
  "[0.1,0.1,0.1]_stdDev_0.1"/1(Signal 1) -> [p6x]
  "[0.1,0.1,0.1]_stdDev_0.1"/3(Signal 3) -> [p6z]
  "[0.1,0.1,0.1]_stdDev_0.1"/2(Signal 2) -> [p6y]
  Clock/1 -> Switch18/2, Switch17/2, Switch16/2, Switch15/2, Switch12/2, Switch13/2, Switch14/2, Switch11/2, Switch10/2, Switch9/2, Switch8/2, Switch7/2, Switch6/2, Switch2/2, Switch1/2, Switch/2, Switch5/2, Switch4/2, Switch3/2
  Switch15/1 -> [vwx_mean]
  Switch16/1 -> [vwy_mean]
  Switch17/1 -> [vwz_mean]
  Moderate/1 -> Switch18/3
  Light/1 -> Switch18/1
  Switch18/1 -> Manual Switch/2

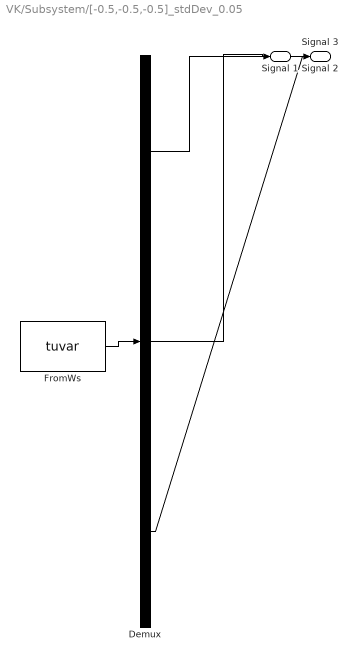
== system VK/Subsystem/[-0.5,-0.5,-0.5]_stdDev_0.05 ==
  Demux : Demux  Tag=STV Demux  Outputs=3
      settings: DisplayOption=none
  FromWs : FromWorkspace  Tag=STV FromWs  VariableName=tuvar
      SigBuilderData=|
      | common.afterFinalStr = 'Extrapolate'
      | common.sampleTime = 0
      | dataSet.timeRange = [0 250]
      | dataSet.name = 'Group 1'
      | sbobj.Groups.Name = 'Group 1'
      | sbobj.Groups.Signals(1).Name = 'Signal 1'
      | sbobj.Groups.Signals(1).XData = [0 0.1 0.2 0.3 0.4 0.5 0.6 0.7 0.8 0.9 1 1.1 ... (2501 elements, 1x2501)]
      | sbobj.Groups.Signals(1).YData = [0.569694957357 0.436090307498 0.4986976519 0.553720899812 0.42639185237 0.379756632794 0.446838716984 0.48684070728 0.569028310643 0.546895103568 0.55040682615 0.39438869238 ... (2501 elements, 1x2501)]
      | sbobj.Groups.Signals(2).Name = 'Signal 2'
      | sbobj.Groups.Signals(2).XData = [0 0.1 0.2 0.3 0.4 0.5 0.6 0.7 0.8 0.9 1 1.1 ... (2501 elements, 1x2501)]
      | sbobj.Groups.Signals(2).YData = [-0.522259216991 -0.494676903771 -0.586695716333 -0.41210712996 -0.520131650712 -0.438112556992 -0.438064112977 -0.513205070505 -0.571016295853 -0.50499228694 -0.453590833493 -0.545173240926 ... (2501 elements, 1x2501)]
      | sbobj.Groups.Signals(3).Name = 'Signal 3'
      | sbobj.Groups.Signals(3).XData = [0 0.1 0.2 0.3 0.4 0.5 0.6 0.7 0.8 0.9 1 1.1 ... (2501 elements, 1x2501)]
      | sbobj.Groups.Signals(3).YData = [-0.493264670056 -0.413778400107 -0.486034561675 -0.466082727071 -0.417330205491 -0.461208246005 -0.376756074939 -0.561287843402 -0.563003572585 -0.439411181906 -0.524417425183 -0.497325198694 ... (2501 elements, 1x2501)]
      | sbobj.Groups.TimeRange = [0 250]
  Signal 1 : Outport  Tag=STV Outport
  Signal 2 : Outport  Tag=STV Outport  Port=2
  Signal 3 : Outport  Tag=STV Outport  Port=3
  wires:
  Demux/1 -> Signal 1/1
  FromWs/1 -> Demux/1
  Demux/2 -> Signal 2/1
  Demux/3 -> Signal 3/1

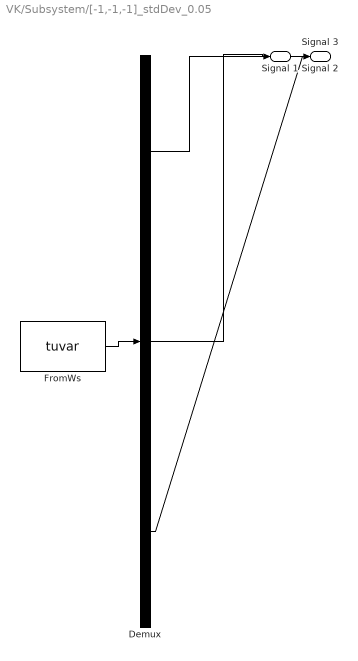
== system VK/Subsystem/[-1,-1,-1]_stdDev_0.05 ==
  Demux : Demux  Tag=STV Demux  Outputs=3
      settings: DisplayOption=none
  FromWs : FromWorkspace  Tag=STV FromWs  VariableName=tuvar
      SigBuilderData=|
      | common.afterFinalStr = 'Extrapolate'
      | common.sampleTime = 0
      | dataSet.timeRange = [0 250]
      | dataSet.name = 'Group 1'
      | sbobj.Groups.Name = 'Group 1'
      | sbobj.Groups.Signals(1).Name = 'Signal 1'
      | sbobj.Groups.Signals(1).XData = [0 0.1 0.2 0.3 0.4 0.5 0.6 0.7 0.8 0.9 1 1.1 ... (2501 elements, 1x2501)]
      | sbobj.Groups.Signals(1).YData = [-1.0187257175 -1.04471262039 -0.985982327884 -1.02191277933 -0.930372602907 -1.0183688747 -1.03977134466 -1.0109199059 -0.945900102419 -1.02834991331 -1.00477496922 -1.07389880766 ... (2501 elements, 1x2501)]
      | sbobj.Groups.Signals(2).Name = 'Signal 2'
      | sbobj.Groups.Signals(2).XData = [0 0.1 0.2 0.3 0.4 0.5 0.6 0.7 0.8 0.9 1 1.1 ... (2501 elements, 1x2501)]
      | sbobj.Groups.Signals(2).YData = [-1.08740482171 -0.969288637631 -1.03742556839 -1.06229290827 -0.933802112069 -0.976516696769 -0.997406868885 -0.991691139389 -0.915226402216 -1.02593546903 -1.02916939104 -1.08180729442 ... (2501 elements, 1x2501)]
      | sbobj.Groups.Signals(3).Name = 'Signal 3'
      | sbobj.Groups.Signals(3).XData = [0 0.1 0.2 0.3 0.4 0.5 0.6 0.7 0.8 0.9 1 1.1 ... (2501 elements, 1x2501)]
      | sbobj.Groups.Signals(3).YData = [-0.982757021998 -0.986951540112 -0.875673379441 -0.930395926116 -0.970570797732 -0.946419196924 -1.01235425602 -1.08763997487 -0.944062620496 -0.993592714808 -0.920152241292 -0.949660629378 ... (2501 elements, 1x2501)]
      | sbobj.Groups.TimeRange = [0 250]
  Signal 1 : Outport  Tag=STV Outport
  Signal 2 : Outport  Tag=STV Outport  Port=2
  Signal 3 : Outport  Tag=STV Outport  Port=3
  wires:
  Demux/3 -> Signal 3/1
  Demux/2 -> Signal 2/1
  FromWs/1 -> Demux/1
  Demux/1 -> Signal 1/1

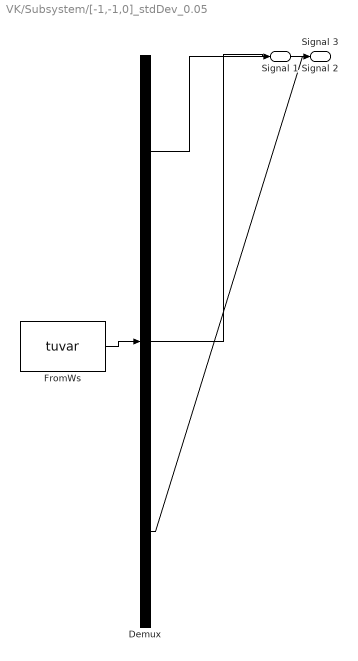
== system VK/Subsystem/[-1,-1,0]_stdDev_0.05 ==
  Demux : Demux  Tag=STV Demux  Outputs=3
      settings: DisplayOption=none
  FromWs : FromWorkspace  Tag=STV FromWs  VariableName=tuvar
      SigBuilderData=|
      | common.afterFinalStr = 'Extrapolate'
      | common.sampleTime = 0
      | dataSet.timeRange = [0 250]
      | dataSet.name = 'Group 1'
      | sbobj.Groups.Name = 'Group 1'
      | sbobj.Groups.Signals(1).Name = 'Signal 1'
      | sbobj.Groups.Signals(1).XData = [0 0.1 0.2 0.3 0.4 0.5 0.6 0.7 0.8 0.9 1 1.1 ... (2501 elements, 1x2501)]
      | sbobj.Groups.Signals(1).YData = [-1.03444798524 -1.00833016999 -0.967319690598 -0.933064368817 -1.01946769932 -1.10139388731 -0.903611258372 -1.05565013836 -1.04339908906 -0.940178016046 -0.982767052937 -1.03992447572 ... (2501 elements, 1x2501)]
      | sbobj.Groups.Signals(2).Name = 'Signal 2'
      | sbobj.Groups.Signals(2).XData = [0 0.1 0.2 0.3 0.4 0.5 0.6 0.7 0.8 0.9 1 1.1 ... (2501 elements, 1x2501)]
      | sbobj.Groups.Signals(2).YData = [-1.04348875365 -1.00533534418 -1.06613744795 -0.953304899774 -0.992021906981 -0.91165467959 -1.04801213466 -0.972390266167 -1.01783668448 -0.989903952671 -1.0379023843 -0.920121224637 ... (2501 elements, 1x2501)]
      | sbobj.Groups.Signals(3).Name = 'Signal 3'
      | sbobj.Groups.Signals(3).XData = [0 0.1 0.2 0.3 0.4 0.5 0.6 0.7 0.8 0.9 1 1.1 ... (2501 elements, 1x2501)]
      | sbobj.Groups.Signals(3).YData = [-0.00561508758574 0.041812930842 0.0728541815851 0.109941329314 -0.0168631555846 0.0730590972983 -0.09068480923 -0.0152448625936 -0.0585171982345 0.121961617828 -0.0599952031419 -0.0448658996061 ... (2501 elements, 1x2501)]
      | sbobj.Groups.TimeRange = [0 250]
  Signal 1 : Outport  Tag=STV Outport
  Signal 2 : Outport  Tag=STV Outport  Port=2
  Signal 3 : Outport  Tag=STV Outport  Port=3
  wires:
  Demux/1 -> Signal 1/1
  FromWs/1 -> Demux/1
  Demux/2 -> Signal 2/1
  Demux/3 -> Signal 3/1

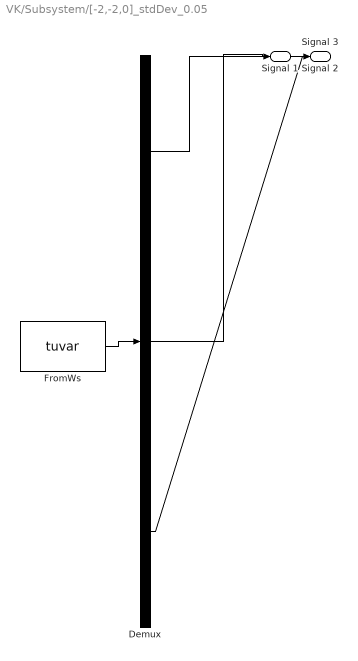
== system VK/Subsystem/[-2,-2,0]_stdDev_0.05 ==
  Demux : Demux  Tag=STV Demux  Outputs=3
      settings: DisplayOption=none
  FromWs : FromWorkspace  Tag=STV FromWs  VariableName=tuvar
      SigBuilderData=|
      | common.afterFinalStr = 'Extrapolate'
      | common.sampleTime = 0
      | dataSet.timeRange = [0 250]
      | dataSet.name = 'Group 1'
      | sbobj.Groups.Name = 'Group 1'
      | sbobj.Groups.Signals(1).Name = 'Signal 1'
      | sbobj.Groups.Signals(1).XData = [0 0.1 0.2 0.3 0.4 0.5 0.6 0.7 0.8 0.9 1 1.1 ... (2501 elements, 1x2501)]
      | sbobj.Groups.Signals(1).YData = [-1.99986539986 -1.94226568431 -1.98391657864 -2.06781483389 -2.00920587634 -1.96736405717 -1.99995499745 -1.99119433191 -1.98654705714 -2.01195847527 -2.03436711043 -2.09265203254 ... (2501 elements, 1x2501)]
      | sbobj.Groups.Signals(2).Name = 'Signal 2'
      | sbobj.Groups.Signals(2).XData = [0 0.1 0.2 0.3 0.4 0.5 0.6 0.7 0.8 0.9 1 1.1 ... (2501 elements, 1x2501)]
      | sbobj.Groups.Signals(2).YData = [-1.92709702467 -1.99434998484 -2.07248718344 -2.00476368434 -1.97066424895 -2.06613967442 -2.18668514075 -2.03502748395 -1.99302153542 -2.06140467568 -2.01160147484 -2.00332753563 ... (2501 elements, 1x2501)]
      | sbobj.Groups.Signals(3).Name = 'Signal 3'
      | sbobj.Groups.Signals(3).XData = [0 0.1 0.2 0.3 0.4 0.5 0.6 0.7 0.8 0.9 1 1.1 ... (2501 elements, 1x2501)]
      | sbobj.Groups.Signals(3).YData = [-0.00561508758574 0.041812930842 0.0728541815851 0.109941329314 -0.0168631555846 0.0730590972983 -0.09068480923 -0.0152448625936 -0.0585171982345 0.121961617828 -0.0599952031419 -0.0448658996061 ... (2501 elements, 1x2501)]
      | sbobj.Groups.TimeRange = [0 250]
  Signal 1 : Outport  Tag=STV Outport
  Signal 2 : Outport  Tag=STV Outport  Port=2
  Signal 3 : Outport  Tag=STV Outport  Port=3
  wires:
  Demux/3 -> Signal 3/1
  Demux/2 -> Signal 2/1
  FromWs/1 -> Demux/1
  Demux/1 -> Signal 1/1

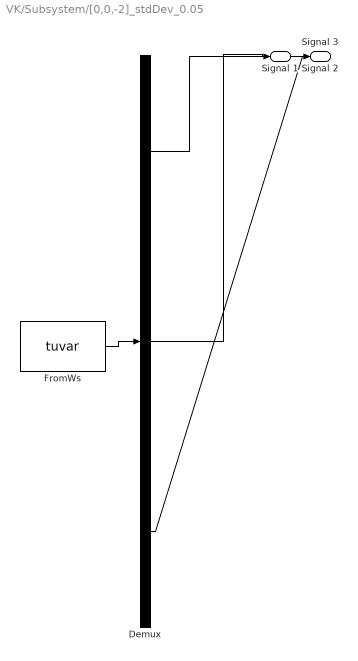
== system VK/Subsystem/[0,0,-2]_stdDev_0.05 ==
  Demux : Demux  Tag=STV Demux  Outputs=3
      settings: DisplayOption=none
  FromWs : FromWorkspace  Tag=STV FromWs  VariableName=tuvar
      SigBuilderData=|
      | common.afterFinalStr = 'Extrapolate'
      | common.sampleTime = 0
      | dataSet.timeRange = [0 250]
      | dataSet.name = 'Group 1'
      | sbobj.Groups.Name = 'Group 1'
      | sbobj.Groups.Signals(1).Name = 'Signal 1'
      | sbobj.Groups.Signals(1).XData = [0 0.1 0.2 0.3 0.4 0.5 0.6 0.7 0.8 0.9 1 1.1 ... (2501 elements, 1x2501)]
      | sbobj.Groups.Signals(1).YData = [0.0268833569773 0.0916942507298 -0.11294234305 0.0431086660184 0.0159382619929 -0.0653844148153 -0.0216796011153 0.0171312233269 0.178919846986 0.138471851494 -0.0674943470078 0.151746173317 ... (2501 elements, 1x2501)]
      | sbobj.Groups.Signals(2).Name = 'Signal 2'
      | sbobj.Groups.Signals(2).XData = [0 0.1 0.2 0.3 0.4 0.5 0.6 0.7 0.8 0.9 1 1.1 ... (2501 elements, 1x2501)]
      | sbobj.Groups.Signals(2).YData = [0.00247173237694 0.053902293741 0.0154089379991 0.0149819271351 -0.00986092277709 -0.00732112164714 -0.00515354348895 -0.139949097292 0.0196637588023 0.0495123576326 -0.0648816455336 -0.0760984181019 ... (2501 elements, 1x2501)]
      | sbobj.Groups.Signals(3).Name = 'Signal 3'
      | sbobj.Groups.Signals(3).XData = [0 0.1 0.2 0.3 0.4 0.5 0.6 0.7 0.8 0.9 1 1.1 ... (2501 elements, 1x2501)]
      | sbobj.Groups.Signals(3).YData = [-1.95370158092 -1.99972447959 -2.03172454264 -1.95708367326 -2.02403882233 -1.92551463965 -2.03146956033 -2.02969753782 -2.03143470204 -1.98218741752 -1.93474571086 -1.98171627744 ... (2501 elements, 1x2501)]
      | sbobj.Groups.TimeRange = [0 250]
  Signal 1 : Outport  Tag=STV Outport
  Signal 2 : Outport  Tag=STV Outport  Port=2
  Signal 3 : Outport  Tag=STV Outport  Port=3
  wires:
  Demux/3 -> Signal 3/1
  Demux/2 -> Signal 2/1
  FromWs/1 -> Demux/1
  Demux/1 -> Signal 1/1

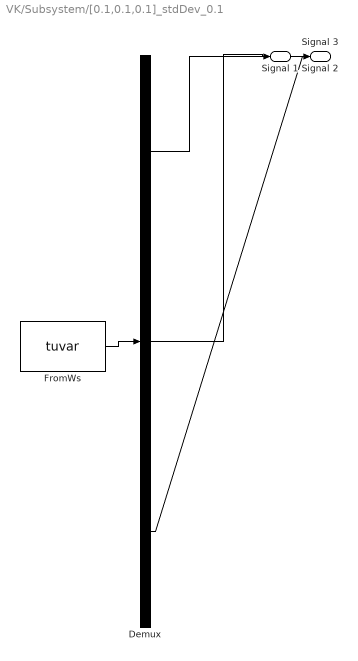
== system VK/Subsystem/[0.1,0.1,0.1]_stdDev_0.1 ==
  Demux : Demux  Tag=STV Demux  Outputs=3
      settings: DisplayOption=none
  FromWs : FromWorkspace  Tag=STV FromWs  VariableName=tuvar
      SigBuilderData=|
      | common.afterFinalStr = 'Extrapolate'
      | common.sampleTime = 0
      | dataSet.timeRange = [0 250]
      | dataSet.name = 'Group 1'
      | sbobj.Groups.Name = 'Group 1'
      | sbobj.Groups.Signals(1).Name = 'Signal 1'
      | sbobj.Groups.Signals(1).XData = [0 0.1 0.2 0.3 0.4 0.5 0.6 0.7 0.8 0.9 1 1.1 ... (2501 elements, 1x2501)]
      | sbobj.Groups.Signals(1).YData = [0.0969080211951 0.0597346376218 0.140031365881 0.135830171431 0.0493595113224 0.071975162971 0.0801893954037 0.1328326758 0.157852008489 0.137448119924 0.0632938495392 -0.000420919255827 ... (2501 elements, 1x2501)]
      | sbobj.Groups.Signals(2).Name = 'Signal 2'
      | sbobj.Groups.Signals(2).XData = [0 0.1 0.2 0.3 0.4 0.5 0.6 0.7 0.8 0.9 1 1.1 ... (2501 elements, 1x2501)]
      | sbobj.Groups.Signals(2).YData = [0.031089718078 0.120637735254 0.0887582721729 0.13240279165 0.0233865902117 0.0763084869599 0.0811838172634 0.118271318563 0.221261659336 0.0828013266296 0.123981093044 0.0952672559137 ... (2501 elements, 1x2501)]
      | sbobj.Groups.Signals(3).Name = 'Signal 3'
      | sbobj.Groups.Signals(3).XData = [0 0.1 0.2 0.3 0.4 0.5 0.6 0.7 0.8 0.9 1 1.1 ... (2501 elements, 1x2501)]
      | sbobj.Groups.Signals(3).YData = [0.168230658419 0.0835392321715 0.123295218736 0.0556297745278 0.17666650755 0.140672847067 0.110955165168 0.0540918679781 0.119339994489 0.132271015304 0.0728934896114 0.0667152231229 ... (2501 elements, 1x2501)]
      | sbobj.Groups.TimeRange = [0 250]
  Signal 1 : Outport  Tag=STV Outport
  Signal 2 : Outport  Tag=STV Outport  Port=2
  Signal 3 : Outport  Tag=STV Outport  Port=3
  wires:
  Demux/1 -> Signal 1/1
  FromWs/1 -> Demux/1
  Demux/2 -> Signal 2/1
  Demux/3 -> Signal 3/1

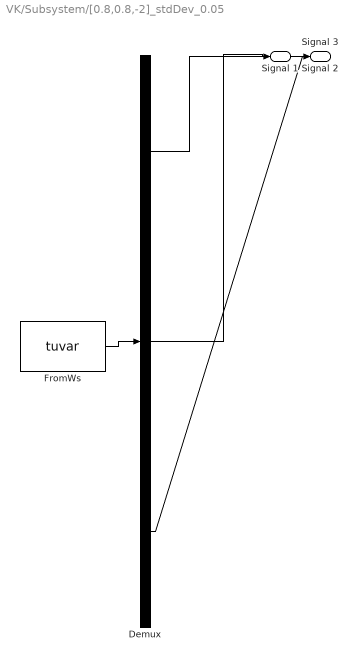
== system VK/Subsystem/[0.8,0.8,-2]_stdDev_0.05 ==
  Demux : Demux  Tag=STV Demux  Outputs=3
      settings: DisplayOption=none
  FromWs : FromWorkspace  Tag=STV FromWs  VariableName=tuvar
      SigBuilderData=|
      | common.afterFinalStr = 'Extrapolate'
      | common.sampleTime = 0
      | dataSet.timeRange = [0 250]
      | dataSet.name = 'Group 1'
      | sbobj.Groups.Name = 'Group 1'
      | sbobj.Groups.Signals(1).Name = 'Signal 1'
      | sbobj.Groups.Signals(1).XData = [0 0.1 0.2 0.3 0.4 0.5 0.6 0.7 0.8 0.9 1 1.1 ... (2501 elements, 1x2501)]
      | sbobj.Groups.Signals(1).YData = [0.789667304647 0.81267106792 0.796948870436 0.753053258875 0.79303402407 0.782538679969 0.808622586827 0.820098003837 0.873696368609 0.790013046454 0.803222941943 0.694802264659 ... (2501 elements, 1x2501)]
      | sbobj.Groups.Signals(2).Name = 'Signal 2'
      | sbobj.Groups.Signals(2).XData = [0 0.1 0.2 0.3 0.4 0.5 0.6 0.7 0.8 0.9 1 1.1 ... (2501 elements, 1x2501)]
      | sbobj.Groups.Signals(2).YData = [0.865278506711 0.740734201684 0.779285057863 0.836235511511 0.766112571103 0.783958215279 0.881832053531 0.682308898216 0.79339348095 0.854579388277 0.766298390198 0.782739521228 ... (2501 elements, 1x2501)]
      | sbobj.Groups.Signals(3).Name = 'Signal 3'
      | sbobj.Groups.Signals(3).XData = [0 0.1 0.2 0.3 0.4 0.5 0.6 0.7 0.8 0.9 1 1.1 ... (2501 elements, 1x2501)]
      | sbobj.Groups.Signals(3).YData = [-2.02213543097 -2.0171078388 -2.01893869928 -2.02912381998 -1.9789127519 -2.00037869882 -1.99343016797 -2.03023854991 -1.9007791937 -1.95354427652 -1.96478483984 -2.00595193734 ... (2501 elements, 1x2501)]
      | sbobj.Groups.TimeRange = [0 250]
  Signal 1 : Outport  Tag=STV Outport
  Signal 2 : Outport  Tag=STV Outport  Port=2
  Signal 3 : Outport  Tag=STV Outport  Port=3
  wires:
  Demux/1 -> Signal 1/1
  FromWs/1 -> Demux/1
  Demux/2 -> Signal 2/1
  Demux/3 -> Signal 3/1

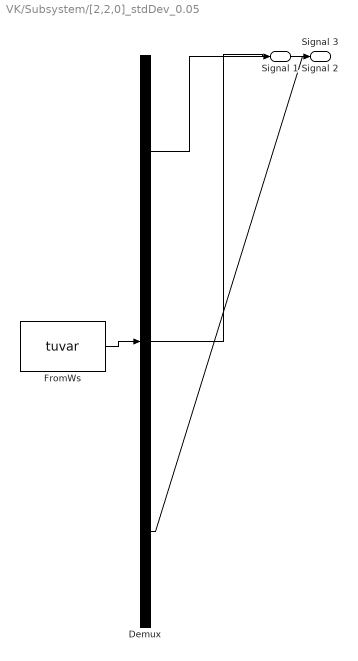
== system VK/Subsystem/[2,2,0]_stdDev_0.05 ==
  Demux : Demux  Tag=STV Demux  Outputs=3
      settings: DisplayOption=none
  FromWs : FromWorkspace  Tag=STV FromWs  VariableName=tuvar
      SigBuilderData=|
      | common.afterFinalStr = 'Extrapolate'
      | common.sampleTime = 0
      | dataSet.timeRange = [0 250]
      | dataSet.name = 'Group 1'
      | sbobj.Groups.Name = 'Group 1'
      | sbobj.Groups.Signals(1).Name = 'Signal 1'
      | sbobj.Groups.Signals(1).XData = [0 0.1 0.2 0.3 0.4 0.5 0.6 0.7 0.8 0.9 1 1.1 ... (2501 elements, 1x2501)]
      | sbobj.Groups.Signals(1).YData = [2.01397381422 2.0654103259 2.04787453947 2.01051344493 2.06767005142 1.99429589857 2.0273027778 1.92231116226 1.93890186291 2.03826130793 1.98229491773 1.97949143589 ... (2501 elements, 1x2501)]
      | sbobj.Groups.Signals(2).Name = 'Signal 2'
      | sbobj.Groups.Signals(2).XData = [0 0.1 0.2 0.3 0.4 0.5 0.6 0.7 0.8 0.9 1 1.1 ... (2501 elements, 1x2501)]
      | sbobj.Groups.Signals(2).YData = [2.00386228398 2.01878037251 2.01977820847 1.99437504555 1.90854816489 2.10457260967 2.01795465611 1.96028276265 1.98863441797 2.07969106774 2.00776028169 2.00892978145 ... (2501 elements, 1x2501)]
      | sbobj.Groups.Signals(3).Name = 'Signal 3'
      | sbobj.Groups.Signals(3).XData = [0 0.1 0.2 0.3 0.4 0.5 0.6 0.7 0.8 0.9 1 1.1 ... (2501 elements, 1x2501)]
      | sbobj.Groups.Signals(3).YData = [0.0134299422824 0.0512037585052 -0.00168838997908 -0.104539612714 -0.0158029639816 0.00664680686666 -0.0332514376645 -0.00233756920818 -0.07521221003 -0.0336663474628 -0.0400204151392 -0.0114102499889 ... (2501 elements, 1x2501)]
      | sbobj.Groups.TimeRange = [0 250]
  Signal 1 : Outport  Tag=STV Outport
  Signal 2 : Outport  Tag=STV Outport  Port=2
  Signal 3 : Outport  Tag=STV Outport  Port=3
  wires:
  Demux/1 -> Signal 1/1
  FromWs/1 -> Demux/1
  Demux/2 -> Signal 2/1
  Demux/3 -> Signal 3/1

== matlab function VK/Subsystem/MATLAB Function1 ==
  data: y output; z input
function y = fcn(z)

y = z/((0.177 + 0.000823*z)^1.2);

== matlab function VK/Subsystem/MATLAB Function ==
  data: Sw input; y output; z input
function y = fcn(Sw,z)

y = Sw/((0.177 + 0.000823*z)^0.4);
